simulink model "sampleModel1709"  (R2023a)
settings: Solver=VariableStepAuto  StartTime=0.0  StopTime=10.0  RelTol=1e-3
libraries: hdlsllib x4, simulink x2
settings Model: Creator=user1  LastModifiedBy=user1

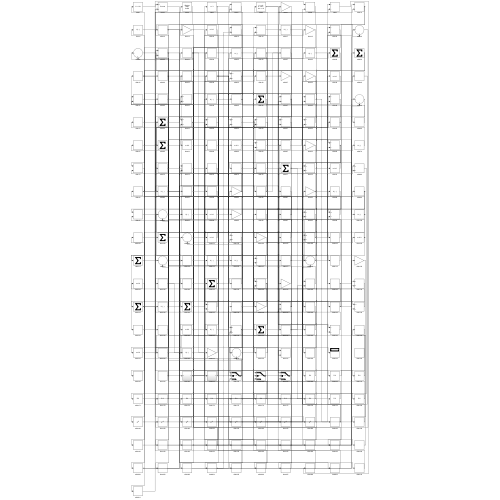
[thumbnail: Simulink's stored preview of the top-level diagram]
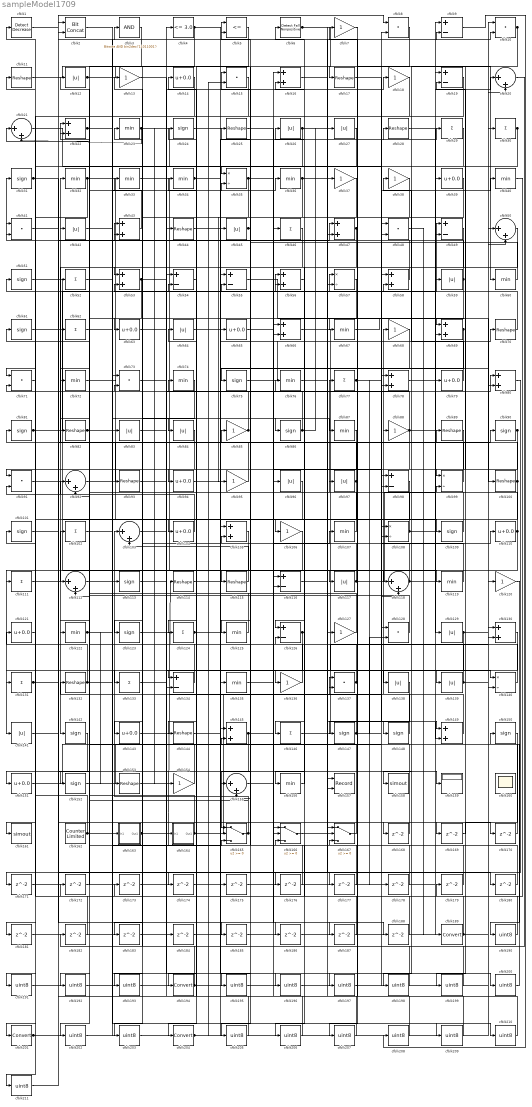
== system sampleModel1709 ==
  cfblk1 : simulink/Logic and Bit Operations/Detect Decrease  vinit=0.0  OutDataTypeStr=boolean
      settings: LibrarySourceBlock=|
      | hdlsllib/Logic and Bit
      | Operations/Detect
      | Decrease
  cfblk{8,10,15,41,48,71,73,91,128,137} (10 alike) : DotProduct  OutDataTypeStr=Inherit: Inherit via internal rule
  cfblk{11,17,25,28,44,70,82,89,93,100,114..115,132,144,153} (15 alike) : Reshape
  cfblk{24,31,51,61,75,81,86,90,101,109,113,123,142,147..148,150,152} (17 alike) : Signum
  cfblk{29..30,46,52,62,77,102,111,124,131,133,146} (12 alike) : Sum  Inputs=+
  cfblk{20..21,50,92,103,112,118,155} (8 alike) : Sum  Inputs=|++
  cfblk{14,39,63,65,79,94,104,110,121,143,151} (11 alike) : Bias  Bias=0.0  SaturateOnIntegerOverflow=off
  cfblk{16,22,43,47,53,56,58,66,69,78,80,105,130,145,149} (15 alike) : Sum
  cfblk{7,13,18,37..38,68,85,88,95,106,120,127,136,154} (14 alike) : Gain
  cfblk{23,32..34,36,40,60,67,72,74,76,87,107,119,122,125,135,156} (18 alike) : MinMax
  cfblk{35,57,99,108,140} (5 alike) : Product  Inputs=*/  RndMeth=Zero  SaturateOnIntegerOverflow=on
  cfblk{9,19,49,54..55,98,116,126,134} (9 alike) : Sum  Inputs=+-
  cfblk{12,26..27,42,45,59,64,83..84,96..97,117,129,138..139,141} (16 alike) : Abs  SaturateOnIntegerOverflow=off
  cfblk157 : Record  FileSettingsInternal="{\"entries\":[{\"content\":{\"excelSettings\":{\"content\":{},\"type\":\"Streamout.ExcelSettings\"}},\"type\":\"Streamout.FileSettingStorage\",\"uuid\":\"\"}],\"packageUris\":[\"http:\\/\\/schema.mathworks.com\\/mf0\\/streamout_blocks\\/R2020a\"],\"version\":\"1.0\"}"  Layout=[1 1]  SignalsInternal="{\"entries\":[{\"content\":{},\"type\":\"RecordBlkView.InputSignals\",\"uuid\":\"\"}],\"packageUris\":[\"http:\\/\\/schema.mathworks.com\\/mf0\\/streamout_blocks\\/R2020a\"],\"version\":\"1.0\"}"  VisualizationBindings="{\"xyplotplugin\":{\"info\":[{\"series\":[{\"bindingParametersList\":[{\"parameter\":\"X-Axis\",\"signalID\":3182,\"signalName\":\"cfblk209\"},{\"parameter\":\"Y-Axis\",\"signalID\":3186,\"signalName\":\"cfblk131\"}],\"seriesID\":12440}],\"subplotID\":1}]}}"  CompatibilityTag=XY  st=-1
  cfblk158 : ToWorkspace  VariableName=simout  SaveFormat=Timeseries  SampleTime=-1
  cfblk159 : Display
  cfblk160 : Scope
      settings: Floating=on
  cfblk161 : ToWorkspace  VariableName=simout  SaveFormat=Timeseries  SampleTime=-1
  cfblk162 : hdlsllib/Sources/Counter Limited  uplimit=7  tsamp=-1
  cfblk163 : Subsystem
      settings: LibrarySourceBlock=|
      | hdlsllib/Ports &
      | Subsystems/Subsystem
  cfblk164 : Subsystem
      settings: LibrarySourceBlock=|
      | hdlsllib/Ports &
      | Subsystems/Subsystem
  cfblk165 : Switch  SaturateOnIntegerOverflow=off  InputSameDT=off
  cfblk166 : Switch  SaturateOnIntegerOverflow=off  InputSameDT=off
  cfblk167 : Switch  SaturateOnIntegerOverflow=off  InputSameDT=off
  cfblk{168..188} (21 alike) : Delay  SampleTime=1
  cfblk{189,194,201,204} (4 alike) : DataTypeConversion  SaturateOnIntegerOverflow=off  RndMeth=Floor
  cfblk{190..193,195..200,202..203,205..211} (19 alike) : DataTypeConversion  OutDataTypeStr=uint8  SaturateOnIntegerOverflow=off  RndMeth=Floor
  cfblk2 : hdlsllib/Logic and Bit Operations/Bit Concat  numInputs=2
  cfblk3 : simulink/Logic and Bit Operations/Bitwise Operator  logicop=AND  UseBitMask=on  BitMask=bin2dec('11011001')  BitMaskRealWorld=Stored Integer
      settings: LibrarySourceBlock=|
      | hdlsllib/Logic and Bit
      | Operations/Bitwise
      | Operator
  cfblk4 : hdlsllib/Logic and Bit Operations/Compare To Constant  relop=<=  const=3.0  OutDataTypeStr=boolean
  cfblk5 : RelationalOperator  Operator=<=  OutDataTypeStr=boolean  InputSameDT=off
  cfblk6 : hdlsllib/Logic and Bit Operations/Detect Fall Nonpositive  vinit=0  OutDataTypeStr=boolean
  wires:
  cfblk165/1 -> cfblk103/1, cfblk92/1
  cfblk163/1(Out1) -> cfblk114/1, cfblk80/1, cfblk57/1
  cfblk33/1 -> cfblk119/1
  cfblk15/1 -> cfblk143/1
  cfblk12/1 -> cfblk95/1, cfblk169/1
  cfblk86/1 -> cfblk27/1, cfblk62/1
  cfblk24/1 -> cfblk55/1
  cfblk149/1 -> cfblk68/1
  cfblk66/1 -> cfblk140/1
  cfblk140/1 -> cfblk64/1
  cfblk10/1 -> cfblk99/1, cfblk198/1
  cfblk116/1 -> cfblk167/1
  cfblk22/1 -> cfblk113/1, cfblk82/1
  cfblk57/1 -> cfblk134/1
  cfblk49/1 -> cfblk142/1
  cfblk123/1 -> cfblk138/1
  cfblk69/1 -> cfblk158/1, cfblk108/2
  cfblk113/1 -> cfblk89/1
  cfblk126/1 -> cfblk174/1, cfblk206/1
  cfblk125/1 -> cfblk51/1
  cfblk122/1 -> cfblk153/1, cfblk200/1
  cfblk47/1 -> cfblk146/1, cfblk57/2
  cfblk50/1 -> cfblk194/1
  cfblk51/1 -> cfblk117/1
  cfblk105/1 -> cfblk141/1
  cfblk42/1 -> cfblk163/1(In1)
  cfblk11/1 -> cfblk17/1
  cfblk30/1 -> cfblk125/1, cfblk118/1
  cfblk162/1 -> cfblk121/1, cfblk165/3
  cfblk32/1 -> cfblk84/1, cfblk181/1
  cfblk111/1 -> cfblk102/1
  cfblk6/1 -> cfblk60/1, cfblk149/2
  cfblk118/1 -> cfblk23/1, cfblk90/1
  cfblk129/1 -> cfblk10/1, cfblk155/2
  cfblk67/1 -> cfblk69/1
  cfblk127/1 -> cfblk81/1
  cfblk143/1 -> cfblk98/1
  cfblk79/1 -> cfblk38/1
  cfblk72/1 -> cfblk109/1
  cfblk147/1 -> cfblk55/2, cfblk110/1, cfblk128/2
  cfblk124/1 -> cfblk70/1, cfblk74/1
  cfblk89/1 -> cfblk156/1
  cfblk28/1 -> cfblk129/1
  cfblk152/1 -> cfblk65/1
  cfblk83/1 -> cfblk136/1
  cfblk90/1 -> cfblk193/1, cfblk205/1
  cfblk56/1 -> cfblk126/1
  cfblk103/1 -> cfblk44/1
  cfblk99/1 -> cfblk32/1
  cfblk84/1 -> cfblk91/1
  cfblk91/1 -> cfblk127/1
  cfblk146/1 -> cfblk30/1
  cfblk64/1 -> cfblk105/1
  cfblk133/1 -> cfblk36/1
  cfblk34/1 -> cfblk80/2, cfblk170/1, cfblk196/1
  cfblk74/1 -> cfblk123/1
  cfblk117/1 -> cfblk39/1, cfblk6/1
  cfblk78/1 -> cfblk79/1
  cfblk154/1 -> cfblk132/1
  cfblk151/1 -> cfblk78/1
  cfblk31/1 -> cfblk3/1, cfblk186/1
  cfblk60/1 -> cfblk15/1
  cfblk106/1 -> cfblk115/1
  cfblk59/1 -> cfblk31/1, cfblk72/1
  cfblk114/1 -> cfblk159/1
  cfblk73/1 -> cfblk4/1
  cfblk135/1 -> cfblk116/2
  cfblk46/1 -> cfblk152/1
  cfblk38/1 -> cfblk133/1
  cfblk141/1 -> cfblk47/1
  cfblk100/1 -> cfblk41/1, cfblk176/1
  cfblk136/1 -> cfblk52/1
  cfblk55/1 -> cfblk100/1
  cfblk156/1 -> cfblk26/1
  cfblk164/1(Out1) -> cfblk137/1, cfblk92/2
  cfblk54/1 -> cfblk204/1
  cfblk139/1 -> cfblk126/2, cfblk99/2, cfblk20/2
  cfblk75/1 -> cfblk37/1
  cfblk97/1 -> cfblk134/2, cfblk14/1, cfblk34/1
  cfblk39/1 -> cfblk144/1
  cfblk81/1 -> cfblk49/1, cfblk5/1
  cfblk19/1 -> cfblk53/1
  cfblk23/1 -> cfblk35/1, cfblk154/1, cfblk21/2
  cfblk134/1 -> cfblk43/1
  cfblk107/1 -> cfblk76/1
  cfblk53/1 -> cfblk112/1, cfblk56/2
  cfblk132/1 -> cfblk83/1, cfblk42/1, cfblk101/1
  cfblk48/1 -> cfblk189/1
  cfblk94/1 -> cfblk59/1
  cfblk70/1 -> cfblk43/2
  cfblk101/1 -> cfblk85/1
  cfblk138/1 -> cfblk147/1
  cfblk109/1 -> cfblk21/1
  cfblk88/1 -> cfblk106/1, cfblk20/1, cfblk11/1
  cfblk3/1 -> cfblk122/1
  cfblk35/1 -> cfblk104/1, cfblk29/1
  cfblk52/1 -> cfblk35/2
  cfblk45/1 -> cfblk75/1, cfblk25/1
  cfblk148/1 -> cfblk22/1
  cfblk85/1 -> cfblk24/1, cfblk73/2
  cfblk121/1 -> cfblk151/1
  cfblk63/1 -> cfblk18/1
  cfblk21/1 -> cfblk78/2
  cfblk110/1 -> cfblk77/1, cfblk155/1
  cfblk43/1 -> cfblk12/1
  cfblk92/1 -> cfblk46/1
  cfblk27/1 -> cfblk71/1
  cfblk4/1 -> cfblk145/1, cfblk183/1
  cfblk137/1 -> cfblk97/1, cfblk5/2
  cfblk95/1 -> cfblk71/2
  cfblk5/1 -> cfblk124/1
  cfblk155/1 -> cfblk107/1
  cfblk71/1 -> cfblk131/1
  cfblk37/1 -> cfblk94/1
  cfblk17/1 -> cfblk149/1
  cfblk115/1 -> cfblk103/2
  cfblk26/1 -> cfblk66/2, cfblk139/1
  cfblk61/1 -> cfblk49/2
  cfblk14/1 -> cfblk111/1
  cfblk65/1 -> cfblk98/2
  cfblk131/1 -> cfblk157/2, cfblk168/1
  cfblk104/1 -> cfblk91/2
  cfblk128/1 -> cfblk61/1
  cfblk1/1 -> cfblk8/1
  cfblk108/1 -> cfblk19/1, cfblk41/2
  cfblk82/1 -> cfblk86/1, cfblk87/1, cfblk165/2
  cfblk58/1 -> cfblk16/2
  cfblk144/1 -> cfblk135/1
  cfblk77/1 -> cfblk40/1, cfblk178/1
  cfblk44/1 -> cfblk28/1
  cfblk8/1 -> cfblk67/1
  cfblk130/1 -> cfblk201/1
  cfblk36/1 -> cfblk10/2, cfblk63/1
  cfblk119/1 -> cfblk56/1
  cfblk167/1 -> cfblk145/2
  cfblk16/1 -> cfblk148/1
  cfblk166/1 -> cfblk58/2
  cfblk112/1 -> cfblk9/2
  cfblk145/1 -> cfblk165/1, cfblk88/1
  cfblk29/1 -> cfblk161/1
  cfblk168/1 -> cfblk53/2
  cfblk169/1 -> cfblk19/2
  cfblk170/1 -> cfblk116/1
  cfblk80/1 -> cfblk171/1
  cfblk171/1 -> cfblk167/2
  cfblk172/1 -> cfblk112/2
  cfblk173/1 -> cfblk8/2
  cfblk174/1 -> cfblk66/1
  cfblk175/1 -> cfblk9/1
  cfblk176/1 -> cfblk166/2
  cfblk41/1 -> cfblk177/1
  cfblk177/1 -> cfblk105/2
  cfblk178/1 -> cfblk22/2
  cfblk40/1 -> cfblk179/1
  cfblk179/1 -> cfblk167/3
  cfblk76/1 -> cfblk180/1
  cfblk180/1 -> cfblk16/1
  cfblk181/1 -> cfblk108/1
  cfblk20/1 -> cfblk182/1
  cfblk182/1 -> cfblk1/1
  cfblk183/1 -> cfblk47/2
  cfblk93/1 -> cfblk184/1
  cfblk184/1 -> cfblk69/2
  cfblk153/1 -> cfblk185/1
  cfblk185/1 -> cfblk140/2
  cfblk186/1 -> cfblk118/2
  cfblk25/1 -> cfblk187/1
  cfblk187/1 -> cfblk166/3
  cfblk62/1 -> cfblk188/1
  cfblk188/1 -> cfblk58/1
  cfblk189/1 -> cfblk172/1, cfblk128/1
  cfblk120/1 -> cfblk190/1
  cfblk190/1 -> cfblk48/1
  cfblk98/1 -> cfblk191/1
  cfblk191/1 -> cfblk48/2
  cfblk96/1 -> cfblk192/1
  cfblk192/1 -> cfblk45/1
  cfblk193/1 -> cfblk96/1
  cfblk194/1 -> cfblk173/1, cfblk33/1, cfblk120/1
  cfblk68/1 -> cfblk195/1
  cfblk195/1 -> cfblk50/1
  cfblk196/1 -> cfblk50/2
  cfblk13/1 -> cfblk197/1
  cfblk197/1 -> cfblk137/2
  cfblk198/1 -> cfblk13/1
  cfblk150/1 -> cfblk199/1
  cfblk199/1 -> cfblk164/1(In1)
  cfblk200/1 -> cfblk150/1
  cfblk201/1 -> cfblk73/1, cfblk93/1
  cfblk87/1 -> cfblk202/1
  cfblk202/1 -> cfblk130/1
  cfblk18/1 -> cfblk203/1
  cfblk203/1 -> cfblk130/2
  cfblk204/1 -> cfblk175/1, cfblk15/2
  cfblk205/1 -> cfblk54/1
  cfblk206/1 -> cfblk54/2
  cfblk7/1 -> cfblk207/1
  cfblk207/1 -> cfblk166/1
  cfblk9/1 -> cfblk208/1
  cfblk208/1 -> cfblk7/1
  cfblk2/1 -> cfblk209/1
  cfblk209/1 -> cfblk157/1
  cfblk102/1 -> cfblk210/1
  cfblk210/1 -> cfblk2/1
  cfblk142/1 -> cfblk211/1
  cfblk211/1 -> cfblk2/2

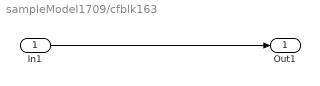
== system sampleModel1709/cfblk163 ==
  In1 : Inport
  Out1 : Outport
  wires:
  In1/1 -> Out1/1

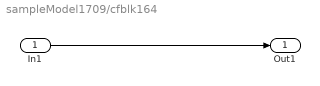
== system sampleModel1709/cfblk164 ==
  In1 : Inport
  Out1 : Outport
  wires:
  In1/1 -> Out1/1
